simulink model "I_PD_C"  (R2017a)
settings: Solver=FixedStepDiscrete  StartTime=0.0  StopTime=Tf  FixedStep=Ts  RelTol=1e-3  EnableMultiTasking=on
values from neighbouring files (symbols this model uses):
  Ts = t(2)-t(1)    [check_filter.m]    (also in closedloop_driver.m = 0.1; openloop_driver.m = 0.1; wheel_parameters.m = 0.05)
libraries: simulink x5
settings Model: Creator=throne  LastModifiedBy=localmgr
settings DataIOCC: LimitDataPoints=on  SaveFormat=Array
settings OptimizationCC: ExpressionDepthLimit=2147483647  InitFltsAndDblsToZero=on  LifeSpan=inf
settings DebuggingCC: UnderspecifiedInitializationDetection=Classic  MergeDetectMultiDrivingBlocksExec=none  SolverPrmCheckMsg=warning  StateNameClashWarn=warning  SFUnexpectedBacktrackingDiag=warning  SFNoUnconditionalDefaultTransitionDiag=warning  SFExecutionAtInitializationDiag=none
settings HardwareCC: ProdBitPerPointer=32  ProdBitPerSizeT=32  ProdBitPerPtrDiffT=32  ProdLargestAtomicFloat=None  ProdIntDivRoundTo=Undefined  ProdEndianess=Unspecified  ProdWordSize=32  ProdHWDeviceType=32-bit Generic
settings ModelReferenceCC: PropagateSignalLabelsOutOfModel=off
settings GRTTargetCC: TargetLangStandard=C89/C90 (ANSI)  GeneratePreprocessorConditionals=Disable all  CombineOutputUpdateFcns=off  GRTInterface=on
settings ConfigComp: CovMetricSettings=dw  CovHtmlReporting=on  CovSaveCumulativeToWorkspaceVar=on  CovSaveSingleToWorkspaceVar=on  CovExternalEMLEnable=off

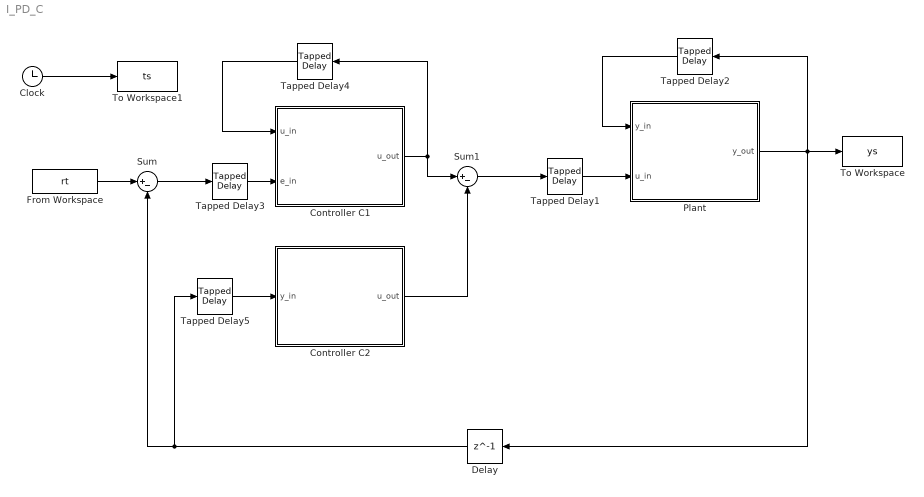
== system I_PD_C ==
  " Controller C1" : MATLAB Function  TreatAsAtomicUnit=on
  " Controller C2" : MATLAB Function  TreatAsAtomicUnit=on
  " Plant" : MATLAB Function  TreatAsAtomicUnit=on
  Clock : Clock
  Delay : Delay  DelayLength=1  InitialCondition=0
  From Workspace : FromWorkspace  VariableName=rt  SampleTime=0
  Sum : Sum  Inputs=|+-
  Sum1 : Sum  Inputs=|+-
  Tapped Delay1 : simulink/Discrete/Tapped Delay  vinit=0.0  samptime=Ts  NumDelays=3  DelayOrder=Newest  includeCurrent=on
  Tapped Delay2 : simulink/Discrete/Tapped Delay  vinit=0.0  samptime=-1  NumDelays=2  DelayOrder=Newest  includeCurrent=on
  Tapped Delay3 : simulink/Discrete/Tapped Delay  vinit=0.0  samptime=Ts  NumDelays=1  DelayOrder=Newest  includeCurrent=on
  Tapped Delay4 : simulink/Discrete/Tapped Delay  vinit=0.0  samptime=-1  NumDelays=1  DelayOrder=Newest  includeCurrent=on
  Tapped Delay5 : simulink/Discrete/Tapped Delay  vinit=0.0  samptime=Ts  NumDelays=1  DelayOrder=Newest  includeCurrent=on
  To Workspace : ToWorkspace  VariableName=ys  SampleTime=-1
  To Workspace1 : ToWorkspace  VariableName=ts  SampleTime=Ts
  wires:
  Clock/1 -> To Workspace1/1
  Tapped Delay2/1 -> " Plant"/1(y_in)
  Tapped Delay1/1 -> " Plant"/2(u_in)
  " Plant"/1(y_out) -> Delay/1, To Workspace/1, Tapped Delay2/1
  " Controller C1"/1(u_out) -> Sum1/1, Tapped Delay4/1
  Tapped Delay4/1 -> " Controller C1"/1(u_in)
  Tapped Delay3/1 -> " Controller C1"/2(e_in)
  From Workspace/1 -> Sum/1
  Sum/1 -> Tapped Delay3/1
  Delay/1 -> Tapped Delay5/1, Sum/2
  Tapped Delay5/1 -> " Controller C2"/1(y_in)
  " Controller C2"/1(u_out) -> Sum1/2
  Sum1/1 -> Tapped Delay1/1

== matlab function I_PD_C/ Controller C1 ==
  data: u_in input size=[1 2]; e_in input size=[1 2]; u_out output
function u_out  = fcn(u_in, e_in)
% This block supports the Embedded MATLAB subset.
% See the help menu for details. 
  u_out = u_in(2)+1.48*e_in(1);

== matlab function I_PD_C/ Plant ==
  data: y_in input size=[1 3]; u_in input size=[1 4]; y_out output
function y_out  = fcn(y_in, u_in)
% This block supports the Embedded MATLAB subset.
% See the help menu for details. 
  y_out = -1*y_in(2)-1*y_in(3)+0.5*u_in(3);

== matlab function I_PD_C/ Controller C2 ==
  data: y_in input size=[1 2]; u_out output
function u_out  = fcn(y_in)
% This block supports the Embedded MATLAB subset.
% See the help menu for details. 
  u_out = 0.057841*(y_in(1) + 0.28*y_in(2));
